simulink model "pos_cont"  (R2014a)
settings: Solver=FixedStepDiscrete  StartTime=0.0  StopTime=inf  FixedStep=sample_time  RelTol=1e-3
undefined symbols (not defined in the file): hip_d, hip_p, hip_sat, leg_d, leg_p, leg_sat, sat_estops
libraries: simulink x1
settings Model: BufferReuse=off  Creator=wmartin  LastModifiedBy=wmartin
settings SolverCC: EnableConcurrentExecution=on
settings DataIOCC: MaxDataPoints=1000000000  SaveFormat=StructureWithTime  SaveOutput=off  SaveTime=off
settings OptimizationCC: BlockReduction=off  OptimizeBlockIOStorage=off  BufferReuse=off  GlobalBufferReuse=off  ExpressionFolding=off  ExpressionDepthLimit=2147483647  LocalBlockOutputs=off  SimCompilerOptimization=On
settings DebuggingCC: UnderspecifiedInitializationDetection=Classic  StateNameClashWarn=warning
settings HardwareCC: ProdIntDivRoundTo=Zero  ProdEndianess=LittleEndian  ProdHWDeviceType=Generic->32-bit x86 compatible
settings ModelReferenceCC: UpdateModelReferenceTargets=IfOutOfDate  ModelReferenceNumInstancesAllowed=Single  ModelReferenceMinAlgLoopOccurrences=on
settings RTWCC: SystemTargetFile=slrt.tlc  TemplateMakefile=slrt_default_tmf  Description=Simulink Real-Time  RTWVerbose=off  ProcessScript=slrt_make_rtw_hook  RTWCompilerOptimization=On
settings SimulinkRealTimeCC: GeneratePreprocessorConditionals=Disable all  EnableShiftOperators=on  RL32LogBufSizeModifier=100000000

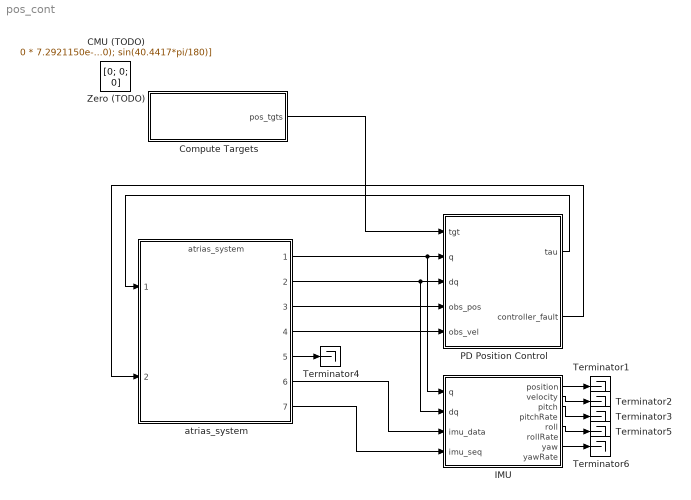
== system pos_cont ==
  Compute Targets : MATLAB Function  TreatAsAtomicUnit=on
  IMU : Subsystem
  PD Position Control : MATLAB Function  TreatAsAtomicUnit=on
  Terminator{1..6} (6 alike) : Terminator
  atrias_system : ModelReference  ModelNameDialog=atrias_system  SimulationMode=Normal  ModelReferenceVersion=1.1696  CopyOfModelName=atrias_system  DefaultDataLogging=on
  CMU (TODO) : Constant  IOType=siggen  Value=0 * 7.2921150e-8 * [0; cos(40.4417*pi/180); sin(40.4417*pi/180)]
  Zero (TODO) : Constant  IOType=siggen  Value=[0; 0; 0]
  wires:
  PD Position Control/1(tau) -> atrias_system/1
  atrias_system/5 -> Terminator4/1
  atrias_system/6 -> IMU/3(imu_data)
  atrias_system/3 -> PD Position Control/4(obs_pos)
  atrias_system/4 -> PD Position Control/5(obs_vel)
  atrias_system/2 -> IMU/2(dq), PD Position Control/3(dq)
  atrias_system/1 -> PD Position Control/2(q), IMU/1(q)
  PD Position Control/2(controller_fault) -> atrias_system/2
  atrias_system/7 -> IMU/4(imu_seq)
  IMU/2(velocity) -> Terminator2/1
  IMU/1(position) -> Terminator1/1
  IMU/3(pitch) -> Terminator3/1
  IMU/5(roll) -> Terminator5/1
  IMU/7(yaw) -> Terminator6/1
  Compute Targets/1(pos_tgts) -> PD Position Control/1(tgt)

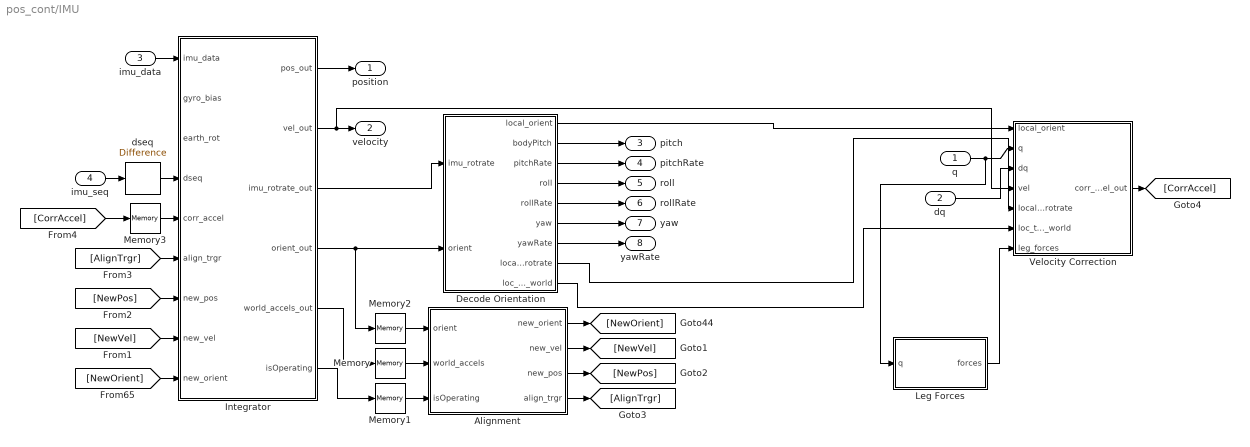
== system pos_cont/IMU ==
  q : Inport
  dq : Inport  Port=2
  imu_data : Inport  Port=3
  imu_seq : Inport  Port=4
  Alignment : MATLAB Function  TreatAsAtomicUnit=on
  Decode Orientation : MATLAB Function  TreatAsAtomicUnit=on
  Integrator : MATLAB Function  TreatAsAtomicUnit=on
  Leg Forces : MATLAB Function  TreatAsAtomicUnit=on
  Memory{,1..3} (4 alike) : Memory
  Velocity Correction : MATLAB Function  TreatAsAtomicUnit=on
  dseq : simulink/Discrete/Difference  ICPrevInput=0.0  InputProcessing=Inherited  OutMin=[]  OutMax=[]  OutDataType=fixdt(1, 16)  OutScaling=2^-10  DoSatur=off
  position : Outport
  velocity : Outport  Port=2
  pitch : Outport  Port=3
  pitchRate : Outport  Port=4
  roll : Outport  Port=5
  rollRate : Outport  Port=6
  yaw : Outport  Port=7
  yawRate : Outport  Port=8
  wires:
  imu_data/1 -> Integrator/1(imu_data)
  Integrator/2(vel_out) -> Velocity Correction/4(vel), velocity/1
  Integrator/1(pos_out) -> position/1
  imu_seq/1 -> dseq/1
  dseq/1 -> Integrator/4(dseq)
  Integrator/5(world_accels_out) -> Memory/1
  Integrator/6(isOperating) -> Memory1/1
  Memory1/1 -> Alignment/3(isOperating)
  Memory/1 -> Alignment/2(world_accels)
  Integrator/4(orient_out) -> Memory2/1, Decode Orientation/2(orient)
  Memory2/1 -> Alignment/1(orient)
  Decode Orientation/2(bodyPitch) -> pitch/1
  Decode Orientation/4(roll) -> roll/1
  Decode Orientation/1(local_orient) -> Velocity Correction/1(local_orient)
  q/1 -> Leg Forces/1(q), Velocity Correction/2(q)
  dq/1 -> Velocity Correction/3(dq)
  Memory3/1 -> Integrator/5(corr_accel)
  Integrator/3(imu_rotrate_out) -> Decode Orientation/1(imu_rotrate)
  Decode Orientation/8(local_rotrate) -> Velocity Correction/5(local_rotrate)
  Decode Orientation/9(loc_to_world) -> Velocity Correction/6(loc_to_world)
  Leg Forces/1(forces) -> Velocity Correction/7(leg_forces)
  Decode Orientation/6(yaw) -> yaw/1
  Decode Orientation/3(pitchRate) -> pitchRate/1
  Decode Orientation/5(rollRate) -> rollRate/1
  Decode Orientation/7(yawRate) -> yawRate/1
  [NewOrient] -> Integrator/9(new_orient)
  Alignment/1(new_orient) -> [NewOrient]
  Alignment/2(new_vel) -> [NewVel]
  [NewVel] -> Integrator/8(new_vel)
  [NewPos] -> Integrator/7(new_pos)
  Alignment/3(new_pos) -> [NewPos]
  Alignment/4(align_trgr) -> [AlignTrgr]
  [AlignTrgr] -> Integrator/6(align_trgr)
  Velocity Correction/1(corr_accel_out) -> [CorrAccel]
  [CorrAccel] -> Memory3/1

== matlab function pos_cont/IMU/Integrator ==
  data: imu_data input double; gyro_bias input double size=3; earth_rot input double size=3; pos_out output; vel_out output double; imu_rotrate_out output; dseq input uint8; orient_out output; sample_time parameter double; corr_accel input; world_accels_out output; isOperating output; align_trgr input; new_pos input size=[3 1]; new_vel input size=[3 1]; new_orient input size=[4 1]
function [pos_out,vel_out,imu_rotrate_out,orient_out,world_accels_out,isOperating] = fcn(imu_data, gyro_bias, earth_rot, dseq, sample_time, corr_accel, align_trgr, new_pos, new_vel, new_orient)
%#codegen

% Local coordinate system: The origin lies at the intersection of the
% lateral and leg rotation axes. X is forward, Z is up, and the coordinate
% system is right-hand (giving a Y axis that points to the robot's left).
%
% IMU coordinate system: The IMU's coordinate axes do not line up with the
% local coordinate system. In the local coordinate system, the IMU's X axis
% points in the [1; 0; -1] direction, the Y axis in the [-1; 0; -1]
% direction, and the Z axis in the [0; 1; 0] direction.
%
% "World" coordinates: Z is up (opposite the gravitational vector), Y is
% locally North (so the Earth's rotation vector lies in the YZ plane), and
% X points locally East.
%
% This block is responsible for maintaining the current location and
% orientation estimates. It outputs a position (in the world coordinate
% system) and an orientation.
%
% The position is in units of meters and is relative to the origin of the
% coordinate system.
%
% The orientation is a rotation quaternion. If applied to the canonical
% basis vectors, it results in the canonical basis vectors of the IMU
% coordinates.
%
% Given a point in IMU coordinates, you could convert that point to the
% world coordinates by first rotating via the orientation quaternion then
% translating by the position vector.
%
% Inputs:
%
%     imu_data   The raw data from the IMU, gyros then accelerometers
%     gyro_bias  The identified gyro bias, as delta radians per cycle (IMU coords)
%     earth_rot  The earth's rotation (rotation vector per cycle, world coordinates)
%     dseq       The change in sequence counter from the previous timestep
%     corr_accel The velocity correction acceleration (m/s/s, world coordinates)
%
% Integration methodology description (the steps in the code are in a
% slightly different order, but the idea is the same):
%
% First, the identified gyro bias is removed from the transmitted delta
% angles value.
%
% Second, the resulting rotation vector is rotated from IMU coordinates
% into world coordinates.
%
% Third, the Earth's rotation vector is removed from the rotation vector.
% This is done using simple vector subtraction, which is a
% (hopefully highly accurate) approximation.
%
% The resulting rotation vector is divided by two to produce an "intermediate"
% rotation vector. This rotation vector as well as the full rotation vector
% are then converted into rotation quaternions.
%
% The incremental and full rotation quaternions are then used to produce
% midpoint and endpoint orientations within the integration step interval.
%
% The three orientation quaternions (previous, midpoint, and new) are used to
% rotate the acceleration samples (linearly interpolated) into the world
% coordinate system, to produce three global acceleration samples.
%
% The gravitational acceleration is then removed from the global
% acceleration samples to produce the true accelerations (note: a rescaling
% is then applied because the IMU outputs in units of g's not m/s^2).
%
% Simpson's rule is then used to integrate the acceleration into positions
% and velocities.

% This system's state
persistent pos          % IMU position (WORLD)
persistent vel          % IMU velocity (WORLD)
persistent orient       % Rotation quaternion from IMU to WORLD
persistent old_accels   % Previous accelerometer readings

% Initialize the position, velocity, and orientation
if isempty(pos) || isempty(vel) || isempty(orient) || isempty(old_accels)
    pos        = [0; 0; 1];
    vel        = zeros(3, 1);
    old_accels = zeros(3, 1);
    % Initialize as level and facing East. Note that this is not a zero
    % rotation quaternion as the IMU's coordinates do not align directly
    % with the local coordinates. We build it up using a series of
    % individual rotations
    orient = rotvecToQuat([-pi/2; 0; 0]); % Rotate about the X axis to align the Z axis w/ the IMU's coordinates.
    orient = quatMult(rotvecToQuat([0; pi/4; 0]), orient); % Rotate 45 degrees to finally align the X and Y axes.
end

% The sequence counter counts module 128. Correct for overflow.
dseq = mod(dseq, 128);

% On the first iteration, reset dcntr to 0, because otherwise it would jump
% to an arbitrary value
persistent isRunning
if isempty(isRunning)
    isRunning = false;
end
if dseq > 0 && ~isRunning
    isRunning = true;
    dseq     = uint8(0);
end

% Counter to determine when to re-normalize the orientation quaternion.
persistent renormCntr
if isempty(renormCntr)
    renormCntr = 0;
end

% Gravitational acceleration: the SI definition of 1 G
gaccel = 9.80665;

% Additional outputs we want to clamp when not processing the IMU data
persistent world_accels
if isempty(world_accels)
    world_accels = [0; 0; gaccel];
end

% If a realignment has been triggered, update the position, velocity, and
% orientation to that computed by the alignment module
if align_trgr
    pos    = new_pos;
    vel    = new_vel;
    orient = new_orient;
end

% Remember this if we didn't just get new data
persistent imu_rotrate
if isempty(imu_rotrate)
    imu_rotrate = zeros(3, 1);
end

% Check if the counter has incremented. If not, then don't update.
if dseq > 0
    % Okay, we've got new data. Do all the processing.

    % Grab the gyro readings and accelerations from the input
    gyros  = imu_data(1:3);
    accels = imu_data(4:6);

    % Remove the gyro bias from the gyro signal
    gyros = gyros - gyro_bias;
    
    % Imu-relative rotation rate
    imu_rotrate = gyros / sample_time;

    % Rotate the gyro readings from the IMU coordinates into the world
    % coordinates
    gyros = quatRot(orient, gyros);

    % Remove the Earth's rotation from the gyro readings
    gyros = gyros - earth_rot;

    % Rescale in case we've missed a cycle. Also compute the delta time for
    % accelerometer integration
    gyros = double(dseq) * gyros;
    dt    = double(dseq) * sample_time;

    % The full and intermediate rotation quaternions
    rot_quat    = rotvecToQuat(gyros);
    midrot_quat = rotvecToQuat(gyros/2);

    % The midpoint and new orientations
    mid_orient = quatMult(midrot_quat, orient);
    new_orient = quatMult(rot_quat,    orient);
    
    % Renormalize the orientation quaternion approximately every 10 seconds
    if renormCntr >= 10000
        renormCntr = 0;
        new_orient = new_orient / norm(new_orient);
    end

    % Sample the accelerations at the beginning, midpoint, and end of the
    % interval
    accel1 = quatRot(orient,     old_accels             );
    accel2 = quatRot(mid_orient, (old_accels + accels)/2);
    accel3 = quatRot(new_orient, accels                 );

    % Update the world-relative sensed acceleration output
    world_accels = gaccel * accel3;

    % Remove the effect of gravity on the accelerations.
    % Note that the accelerations are still in units of G's
    accel1(3) = accel1(3) - 1;
    accel2(3) = accel2(3) - 1;
    accel3(3) = accel3(3) - 1;

    % Rescale the accelerations to units of m/s
    accel1 = accel1 * gaccel;
    accel2 = accel2 * gaccel;
    accel3 = accel3 * gaccel;

    % Execute a second-order version of Simpson's rule to integrate
    % acceleration and velocity into position. Note that the second-order
    % Simpson's rule coefficients look unusual, but they are accurate.
    pos = pos + dt * vel + dt * dt * [accel1 accel2 accel3] * [1; 2; 0]/6;

    % Execute Simpson's Rule to integrate acceleration into velocity,
    % and additionally sum in the correction acceleration
    vel = vel + dt * [accel1 accel2 accel3] * [1; 4; 1] / 6 + dt * corr_accel;

    % Update the old acceleration and orientation values for the next iteration
    orient     = new_orient;
    old_accels = accels;
end

% Last, copy the current position, velocity, and orientation over to the
% outputs
pos_out          = pos;
vel_out          = vel;
orient_out       = orient;
world_accels_out = world_accels;
isOperating      = isRunning;
imu_rotrate_out  = imu_rotrate;

== matlab function pos_cont/PD Position Control ==
  data: tgt input; tau output; q input; dq input; obs_pos input; obs_vel input; hip_sat parameter; leg_sat parameter; leg_p parameter; leg_d parameter; hip_p parameter; hip_d parameter; sat_estops parameter boolean; controller_fault output boolean
function [tau,controller_fault] = fcn(tgt, q, dq, obs_pos, obs_vel, hip_sat, leg_sat, leg_p, leg_d, hip_p, hip_d, sat_estops)
%#codegen

% Grab the motor positions and velocities in the same order as tau
mot_q  = [ obs_pos([1 2])';  q(9)
           obs_pos([3 4])';  q(10) ];
       
mot_dq = [ obs_vel([1 2])'; dq(9)
           obs_vel([3 4])'; dq(10) ];

% Do the control
tau = [leg_p; leg_p; hip_p; leg_p; leg_p; hip_p] .* (tgt - mot_q) - ...
      [leg_d; leg_d; hip_d; leg_d; leg_d; hip_d] .* mot_dq;

% Apply the saturation limits
all_sats  = [leg_sat; leg_sat; hip_sat; leg_sat; leg_sat; hip_sat];
tau_unsat = tau;
tau       = min(tau,  all_sats);
tau       = max(tau, -all_sats);

% Check if any saturations have been hit. If so, then possibly transmit a
% controller fault
controller_fault = sat_estops & any(tau ~= tau_unsat);

== matlab function pos_cont/IMU/Alignment ==
  data: orient input; world_accels input; new_orient output; new_vel output; new_pos output; isOperating input; align_trgr output boolean
function [new_orient,new_vel,new_pos,align_trgr] = fcn(orient, world_accels, isOperating)
%#codegen

% Retain whether or not we're starting up (integrating for the alignment)
persistent isAligning
if isempty(isAligning)
    isAligning = false;
end

% Default outputs. Only set new ones right when alignment finishes
new_orient = orient;
new_vel    = zeros(3, 1);
new_pos    = [0; 0; 1];
align_trgr = false;

% We use this to determine the average acceleration direction.
persistent accels_int
if isempty(accels_int)
    accels_int = zeros(3, 1);
end

% Exit immediately if alignment is complete or operation hasn't begin yet
if ~isAligning || ~isOperating
    return
end

% Integrate the accelerations
accels_int = accels_int + world_accels;

% If world_accels exceeds a tolerance, stop the alignment and compute the
% updates
if norm(accels_int) > 10 * 10 * 1000 % 10 seconds at 10 m/s^2 at 1 kHz
    % Normalize the acceleration vector
    accels_int = accels_int / norm(accels_int);

    % Grab the rotation direction in which to re-orient the orientation
    rot_dir = cross(accels_int, [0; 0; 1]);

    % The magnitude of the necessary correction rotation
    rot_mag = asin(norm(rot_dir));

    % Update the rotation direction to be the correct rotation vector
    rot_dir = rot_mag * rot_dir / norm(rot_dir);

    % Create the update quaternion
    upQuat = rotvecToQuat(rot_dir);

    % Apply the update to the current orientation
    new_orient = quatMult(upQuat, orient);

    % Trigger the integrator to re-align
    align_trgr = true;

    % Shut off the alignment process
    isAligning = false;
end

== matlab function pos_cont/IMU/Decode Orientation ==
  data: imu_rotrate input size=3; orient input size=4; local_orient output size=4; bodyPitch output size=1; pitchRate output; roll output double size=1; rollRate output; yaw output; yawRate output; local_rotrate output size=3; loc_to_world output size=4
function [local_orient,bodyPitch,pitchRate,roll,rollRate,yaw,yawRate,local_rotrate,loc_to_world] = fcn(imu_rotrate,orient)
%#codegen

% This decodes the orientation vector into more useful angles
%
% Returns:
%     local_orient Rotation quaternion: canonical -> local basis

% Create the imu -> local rotation quaternion
% Applying this to a IMU-coordinates vector will produce a local
% coordinates vector.
imu_to_loc = rotvecToQuat([-pi/2; 0; 0]); % Rotate about the X axis to align the Z axis w/ the IMU's coordinates.
imu_to_loc = quatMult(rotvecToQuat([0; pi/4; 0]), imu_to_loc); % Rotate 45 degrees to finally align the X and Y axes.

% Compute the local->world rotation quaternion
loc_to_world = quatMult(orient, quatConj(imu_to_loc));

% Compute the local-coordinates rotation rate from the imu-coordinates
% rotation rate
local_rotrate = quatRot(imu_to_loc, imu_rotrate);

% Also compute the world-relative rotation rate, used for the calculation
% of yaw rate
world_rotrate = quatRot(orient, imu_rotrate);

% Use the imu to location vector to calculate the local orientation
% quaternion
local_orient = quatMult(orient, quatConj(imu_to_loc));

% Next, calculate the pitch. To do this, we rotate the world Z vector into
% the local coordinates. We then project it to the saggital (X-Z) plane and
% use trig to identify the angle.
worldZ_loc = invQuatRot(local_orient, [0; 0; 1]);
bodyPitch  = -atan2(worldZ_loc(1), worldZ_loc(3));

% Differentiate the above formulas to get the pitch rate
worldZ_vel = cross(local_rotrate, worldZ_loc);
pitchRate  = [-worldZ_loc(3), worldZ_loc(1)] * [worldZ_vel(1); worldZ_vel(3)];

% Use the same world Z vector rotation to calculate the roll.
% A roll of 0 indicates ATRIAS is vertical, positive = rolled right
% First, project the Z vector onto the frontal plane, which rotates with
% the robot's pitch (and heading).
% Use complex-step differentiation to differentiate through the quaternion
% rotation.
ssize      = eps^2;
cx_wz_loc  = cxdiff_init(worldZ_loc, worldZ_vel, ssize);
cx_bp      = cxdiff_init(bodyPitch,  pitchRate,  ssize);
cx_wz_loc  = quatRot(rotvecToQuat([0; cx_bp;     0]), cx_wz_loc );
[worldZ_loc, worldZ_vel] = cxdiff_eval(cx_wz_loc, ssize);
%worldZ_loc = quatRot(rotvecToQuat([0; bodyPitch; 0]), worldZ_loc);
roll       = atan2(worldZ_loc(2), worldZ_loc(3));

% Similarly, compute the rolling rate through analytical differentiation
rollRate   = [worldZ_loc(3), -worldZ_loc(2)] * [worldZ_vel(2); worldZ_vel(3)];

% The heading is calculated by projecting the local X direction to the
% world coordinates, then projecting that vector to the X-Y plane and
% computing heading that way. Facing east is a zero heading, going north is
% pi/2
localX_world = quatRot(local_orient, [1; 0; 0]);
yaw          = atan2(localX_world(2), localX_world(1));

% The yaw rate is just the world Z rotation rate
yawRate = world_rotrate(3);

== matlab function pos_cont/IMU/Velocity Correction ==
  data: local_orient input size=4; corr_accel_out output size=3; q input; dq input; vel input size=3; local_rotrate input size=3; loc_to_world input size=4; leg_forces input; HIP_WIDTH parameter size=1
function corr_accel_out  = fcn(local_orient,q,dq,vel,local_rotrate,loc_to_world,leg_forces,HIP_WIDTH)
%#codegen

% Whether or not each leg is on the ground.
% The first element is for the left leg, the second is for the right.
inStance = leg_forces > 100;

% Do everything in parallel -- the left column corresponds with the left
% leg and the right column with the right.

% First, pull the relevant values out of q and dq

% We'll do most of the work in a robot-relative coordinate system.
% After computing the robot-relative toe velocity, we'll use the robot's
% rotation rate and velocity to convert it into world coordinates

% Compute the angular velocity of the hip
w_h = [ dq(10), -dq(9)
        0        0
        0        0    ];

% The "direction" of the hip, which points from the center of the hip's
% rotation out through the axis of rotation of the leg's motors.
d_h = [ 0          0
        cos(q(10)) -cos(q(9))
        sin(q(10))  sin(q(9)) ];

% The positions of the hips
r_h = HIP_WIDTH * d_h;

% Compute the linear velocities of the hips
v_h = cross(w_h, r_h);

% Angular velocity of the topmost leg link endpoint (link B, the front link)
w_b = w_h + d_h * diag([ dq(8), -dq(4) ]);

% Distance between the hips and the corresponding B link endpoints
r_b = .5 * [ sin(q(8))            sin(q(4))
            -sin(q(10))*cos(q(8)) sin(q(9))*cos(q(4))
             cos(q(8))*cos(q(10)) cos(q(4))*cos(q(9)) ];

% Linear velocity of point B (the end of the B segment)
v_b = v_h + cross(w_b, r_b);

% Angular velocity of the toe link
w_a = w_b + d_h * diag([dq(6), -dq(2)]);

% Displacement from the B link endpoint to the toe
r_a = .5 * [ sin(q(6))            sin(q(2))
            -sin(q(10))*cos(q(6)) sin(q(9))*cos(q(2))
             cos(q(10))*cos(q(6)) cos(q(9))*cos(q(2)) ];

% Velocity of the toe
v_a = v_b + cross(w_a, r_a);

% Now adjust the toe velocity to include the torso rotation rate
local_toe_rate = v_a + cross(repmat(local_rotrate,1,2), r_h + r_b + r_a);

% Rotate the velocity into the global coordinates and offset to get the
% world-coordinates kinematic toe rate
kine_vel      = [0 0; 0 0; 0 0];
kine_vel(:,1) = vel + quatRot(loc_to_world, local_toe_rate(:,1));
kine_vel(:,2) = vel + quatRot(loc_to_world, local_toe_rate(:,2));

% Compute the correction acceleration
corr_accel = -1 * kine_vel;

% Zero out the correction acceleration for legs with no ground contact
corr_accel = corr_accel * diag(inStance);

% Sum up the final per-toe correction accelerations to get the final
% (total) correction acceleration
corr_accel_out = sum(corr_accel, 2);

== matlab function pos_cont/IMU/Leg Forces ==
  data: q input; forces output size=[2 1]; k_sea parameter
function forces = fcn(q, k_sea)
%#codegen

% Motor and gear positions (LF, LB, RF, RB)
mot_q = q([8; 6; 4; 2]);
leg_q = q([7; 5; 3; 1]);

% Torques
T = reshape(k_sea(end:-1:1),[],1) .* (mot_q - leg_q);

% Pull out the T1 and T2 torques (for front/back motors)
T1 = T([1 3]);
T2 = T([2 4]);

% Translate to OSU coordinates for the Z force calculation
A1 = mot_q([1 3]) - pi/2;
A2 = mot_q([2 4]) - pi/2;

% Calculate the Z forces for each leg
forces = 2 * csc(A1 - A2) .* (-sin(A2) .* T1 + sin(A1) .* T2);

== matlab function pos_cont/Compute Targets ==
  data: splay_ang parameter; pos_tgts output
function pos_tgts = fcn(splay_ang)
%#codegen

% Do the initial computation in degrees for convenience
pos_tgts = [180; 180; 0; 180; 180; 0] + [1; -1; 0; 1; -1; 0] * splay_ang/2;

% Convert to radians for control
pos_tgts = pos_tgts * pi/180;
